simulink model "blocks"  (R2019a)
settings: Solver=VariableStepAuto  StartTime=0.0  StopTime=10.0  RelTol=1e-3
settings Model: Creator=adeye  LastModifiedBy=adeye

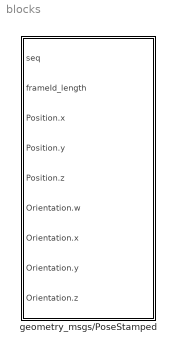
== system blocks ==
  geometry_msgs/PoseStamped : Subsystem  mask{topic='/move_base_simple/goal', message_type='geometry_msgs/PoseStamped', port=9090, timeout=2, frameId='world'}
      mask prompts: topic "Topic name"; message_type "Message type"; timeout "Timeout (s)"

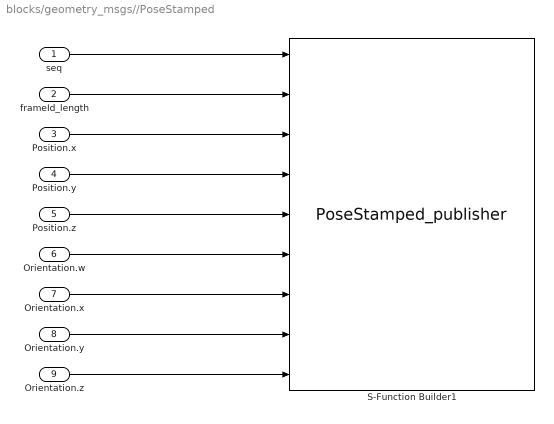
== system blocks/geometry_msgs//PoseStamped ==
  seq : Inport
  frameId_length : Inport  Port=2
  Position.x : Inport  Port=3
  Position.y : Inport  Port=4
  Position.z : Inport  Port=5
  Orientation.w : Inport  Port=6
  Orientation.x : Inport  Port=7
  Orientation.y : Inport  Port=8
  Orientation.z : Inport  Port=9
  S-Function Builder1 : S-Function  InitFcn=try, set_param(gcb,'FunctionName','PoseStamped_publisher'), end  FunctionName=PoseStamped_publisher  Parameters=int8(topic),int8(message_type),port,timeout,uint8(1)  SFunctionModules=PoseStamped_publisher_wrapper rosbridge_functions  SFunctionDeploymentMode=off  EnableBusSupport=off  mask(S-Function Builder){}
      mask help: Simulink:masks:SFunctionBuilder_MD
      mask init:
      | val = [[.9  0.75 0.75 1 1 .9 .9 1]',[1 1 0.75 0.75 .9 .9 1 .9]'];try , sys = get_param(gcb,'SfunBuilderFcnName');if isempty(sys), sys = get_param(gcb,'FunctionName'); end,catch, sys = get_param(gcb,'FunctionName'); end
      settings: CopyFcn=set_param(gcbh,'LinkStatus','none')  PreSaveFcn=try, set_param(gcb,'FunctionName','PoseStamped_publisher'), end  OpenFcn=sfunctionwizard(gcbh)
      mask Display: plot(val(:,1),val(:,2)),disp(sys), port_label('input',1,'seq'), port_label('input',2,'frameId_length'), port_label('input',3,'positionX'), port_label('input',4,'positionY'), port_label('input',5,'positionZ'), port_label('input',6,'orientationW'), port_label('input',7,'orientationX'), port_label('input',8,'orientationY'), port_label('input',9,'orientationZ')
  wires:
  Position.x/1 -> S-Function Builder1/3
  Position.y/1 -> S-Function Builder1/4
  Position.z/1 -> S-Function Builder1/5
  Orientation.w/1 -> S-Function Builder1/6
  Orientation.x/1 -> S-Function Builder1/7
  Orientation.y/1 -> S-Function Builder1/8
  Orientation.z/1 -> S-Function Builder1/9
  seq/1 -> S-Function Builder1/1
  frameId_length/1 -> S-Function Builder1/2
